simulink model "SPENSER_Control_System"  (R2023a)
settings: Solver=VariableStepAuto  StartTime=0.0  StopTime=10  RelTol=1e-3
model workspace: external: MATLAB File C:\Users\Memoh\Desktop\E-Just\Years\Fourth Year\Second Semester\Selected Topics\Projects\Mini-Project_1 Cartesian Robot (SPENCER)\Control System\XML\Spencer_URDF_DataFile.m (data not in the file)
undefined symbols (not defined in the file or in its folder): Kd, Ki, Kp, smiData, X, Y, Z
libraries: sm_lib x35, nesl_utility x12, slpidlib x4
(part 2 of 2)

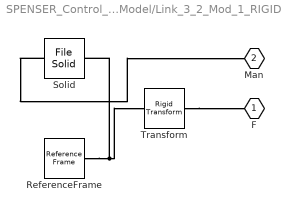
== system SPENSER_Control_System/SPENCER Mechanical Model/Link_3_2_Mod_1_RIGID ==
  ReferenceFrame : sm_lib/Frames and Transforms/Reference Frame
  Solid : sm_lib/Body Elements/File Solid  ExtGeomFileName=S:\Master Portfolio\SPENSER-PID-Control\Software\MATLAB\XML\Link 3_2 Mod_Default_sldprt.STEP  UnitType=FromFile  ExtGeomFileUnits=m  StepReaderType=HEX  ExportConvexHullGeometry=off  InertiaType=Custom  Mass=smiData.Solid(2).mass  MassUnits=kg  CenterOfMass=smiData.Solid(2).CoM  CenterOfMassUnits=mm  MomentsOfInertia=smiData.Solid(2).MoI  MomentsOfInertiaUnits=kg*mm^2  ProductsOfInertia=smiData.Solid(2).PoI  ProductsOfInertiaUnits=kg*mm^2  BasedOnType=DensityFromFile  Density=1000  DensityUnits=kg/m^3  DoExposeReferenceFrame=on  SerializedFrames=<Frames><Frame><Id>Frame1</Id><Value><Name>Manipulator</Name><Origin><Source>GeometricFeature</Source><FeatureName>point 6472</FeatureName></Origin><PrimaryAxis><DefinedDirection>+Z</DefinedDirection><Source>ReferenceFrame</Source><SourceDirection>+Z</SourceDirection><FeatureName></FeatureName></PrimaryAxis><SecondaryAxis><DefinedDirection>+X</DefinedDirection><Source>ReferenceFrame</Source><SourceDirection>+X</SourceDirection><FeatureName></FeatureName></SecondaryAxis></Value></Frame></Frames>  GraphicType=FromGeometry  MarkerShape=Sphere  MarkerSize=10  GraphicVisPropType=SimpleVisualProperties  GraphicDiffuseColor=smiData.Solid(2).color  GraphicSpecularColor=[0.5 0.5 0.5 1.0]  GraphicAmbientColor=[0.15 0.15 0.15 1.0]  GraphicEmissiveColor=[0.0 0.0 0.0 1.0]  GraphicShininess=75  GraphicOpacity=smiData.Solid(2).opacity
  Transform : sm_lib/Frames and Transforms/Rigid Transform  TranslationMethod=Cartesian  TranslationStandardOffset=0  TranslationStandardOffsetUnits=m  TranslationStandardAxis=+Z  TranslationCartesianOffset=smiData.RigidTransform(2).translation  TranslationCartesianOffsetUnits=mm  TranslationROffset=0  TranslationROffsetUnits=m  TranslationZOffset=0  TranslationZOffsetUnits=m  TranslationThetaOffset=0  TranslationThetaOffsetUnits=deg  RotationMethod=ArbitraryAxis  RotationAngleUnits=rad  RotationStandardAxis=+Z  RotationAngle=smiData.RigidTransform(2).angle  RotationArbitraryAxis=smiData.RigidTransform(2).axis  FollAlignAxisA=+X  BaseAlignAxisA=+Y  FollAlignAxisB=+Y  BaseAlignAxisB=+Z  RotationSequenceAxes=FollowerAxes  RotationSequence=XYX  RotationSequenceAngles=[0 0 0]  RotationSequenceAnglesUnits=deg  RotationMatrix=[1 0 0; 0 1 0; 0 0 1]  Quaternion=[1 0 0 0]
  F : PMIOPort  Side=Left
  Man : PMIOPort  Port=2  Side=Left
  connections:
  Solid/RConn1 -- ReferenceFrame/RConn1 -- Transform/LConn1
  Transform/RConn1 -- F/RConn1
  Solid/LConn1 -- Man/RConn1

== matlab function SPENSER_Control_System/Forward Kinematics ==
  data: x output; y output; z output; j1 input; j2 input; j3 input; j4 input
function [x, y, z] = func2(j1, j2, j3, j4)
%{
FUNC2 Calls the "forward_kinematics()" function saved in "Scripts" folder
in project MATLAB directory.
%}

[x, y, z] = forward_kinematics(j1, j2, j3, j4);

end

== matlab function SPENSER_Control_System/Inverse Kinematics ==
  data: xd input; yd input; zd input; des1 output; des2 output; des3 output; des4 output
function [des1, des2, des3, des4] = func1(xd, yd, zd)
%{
FUNC1 Calls the "inverse_kinematics()" function saved in "Scripts" folder
in project MATLAB directory.
%}

[des1, des2, des3, des4] = inverse_kinematics(xd, yd, zd);

end
